simulink model "lin_Model_stdSS"  (R2023b)
settings: Solver=VariableStepAuto  StartTime=0.0  StopTime=10.0  RelTol=1e-3
libraries: cstblocks x2
settings Model: Creator=maxja  LastModifiedBy=maxja

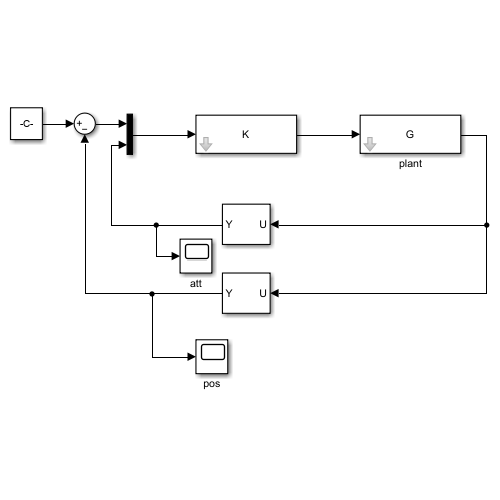
[thumbnail: Simulink's stored preview of the top-level diagram]
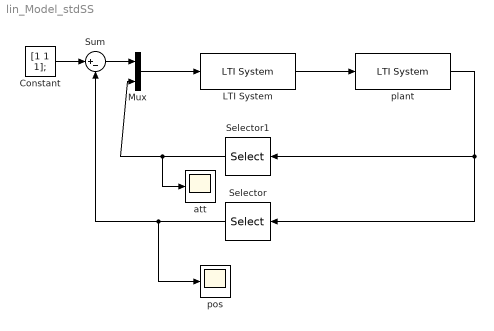
== system lin_Model_stdSS ==
  Constant : Constant  Value=[1 1 1];
  LTI System : cstblocks/LTI System  sys=K  IC=[]  PadeOrder=0
  Mux : Mux  Inputs=2
  Selector : Selector  InputPortWidth=6  IndexOptions=Index vector (dialog)  Indices=[1:3]  OutputSizes=1
  Selector1 : Selector  InputPortWidth=6  IndexOptions=Index vector (dialog)  Indices=[4:6]  OutputSizes=1
  Sum : Sum  Inputs=|+-
  att : Scope
  plant : cstblocks/LTI System  sys=G  IC=[]  PadeOrder=0
  pos : Scope
  wires:
  LTI System/1 -> plant/1
  Constant/1 -> Sum/1
  Sum/1 -> Mux/1
  Mux/1 -> LTI System/1
  plant/1 -> Selector1/1, Selector/1
  Selector1/1 -> att/1, Mux/2
  Selector/1 -> pos/1, Sum/2
